simulink model "DriverModel"  (R2026b)
settings: Solver=ode45  StopTime=Simulation.StopTimeSmoke.Value
undefined symbols (not defined in the file): DefaultDriverCommandBus
settings Model: DataDictionary=VehicleData.sldd  Creator=Xu Dingyi  LastModifiedBy=29358

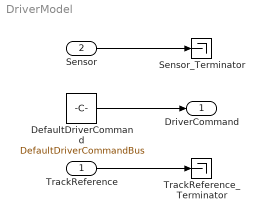
== system DriverModel ==
  TrackReference : Inport  OutDataTypeStr=Bus: TrackReferenceBus
  Sensor : Inport  Port=2  OutDataTypeStr=Bus: SensorBus
  DefaultDriverCommand : Constant  Value=DefaultDriverCommandBus  OutDataTypeStr=Bus: DriverCommandBus  SampleTime=-1
  Sensor_Terminator : Terminator
  TrackReference_Terminator : Terminator
  DriverCommand : Outport  OutDataTypeStr=Bus: DriverCommandBus
  wires:
  DefaultDriverCommand/1 -> DriverCommand/1
  Sensor/1 -> Sensor_Terminator/1
  TrackReference/1 -> TrackReference_Terminator/1
